simulink model "neeew"  (Simulink 8.3)
settings: Solver=ode23tb  SolverMode=SingleTasking  StartTime=0.0  StopTime=1  RelTol=1e-3
undefined symbols (not defined in the file): D1, Delta
libraries: spsThreePhaseVIMeasurementLib x15, spsPiSectionLineLib x15, spsThreePhaseBreakerLib x14, spsThreePhaseParallelRLCLoadLib x5, spsThreePhaseProgrammableVoltageSourceLib x2, spsThreePhaseTransformerTwoWindingsLib x2, spsGroundLib x2, spspowerguiLib x1
settings Model: Creator=DELL  LastModifiedBy=Ayyan LapTop  CovMetricSettings=dwe  CovHtmlReporting=off  covSaveCumulativeToWorkspaceVar=off  CovSaveSingleToWorkspaceVar=off  CovExternalEMLEnable=on  CovSFcnEnable=on
settings SolverCC: ZeroCrossAlgorithm=Adaptive
settings DataIOCC: LimitDataPoints=off  SaveFormat=StructureWithTime  SignalLoggingSaveFormat=Dataset
settings DebuggingCC: UnderspecifiedInitializationDetection=Simplified  MergeDetectMultiDrivingBlocksExec=error  MaxConsecutiveZCsMsg=none  SolverPrmCheckMsg=none  FrameProcessingCompatibilityMsg=error  StateNameClashWarn=none  SFUnexpectedBacktrackingDiag=error  SFNoUnconditionalDefaultTransitionDiag=error
settings HardwareCC: ProdBitPerPointer=64  ProdLargestAtomicFloat=Float  ProdIntDivRoundTo=Zero  ProdEndianess=LittleEndian  ProdHWDeviceType=Specified
settings ModelReferenceCC: PropagateSignalLabelsOutOfModel=on
settings GRTTargetCC: TargetLangStandard=C99 (ISO)  CombineOutputUpdateFcns=on  GRTInterface=off

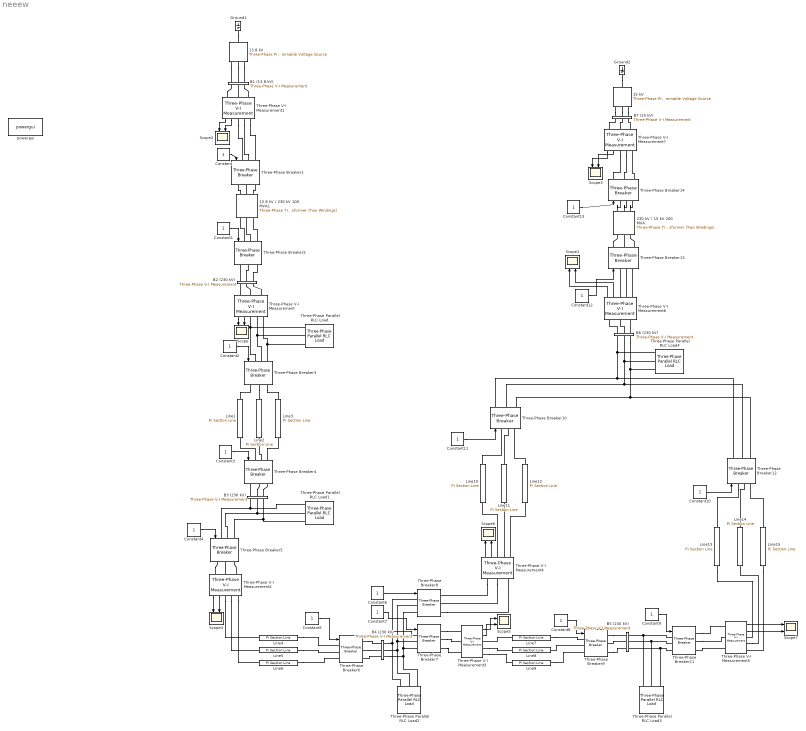
== system neeew ==
  13.8 kV : spsThreePhaseProgrammableVoltageSourceLib/Three-Phase Programmable Voltage Source  PositiveSequence=[13.8e3 0 60]  VariationEntity=Amplitude  VariationType=Table of time-amplitude pairs  VariationTypeAlt=Step  VariationStep=-0.2  VariationRate=10  VariationMagnitude=0.3  VariationFrequency=2  VariationTiming=[0.05 0.05+5/60]  VariationPhaseA=off  Amplitudes=[1 0.75 1.0]  TimeValues=[0 0.03 0.13]  HarmonicGeneration=off  HarmonicA=[1 -0.1 0 2]  HarmonicB=[2 0.15 35 2]*0  Timing="[0.1  2]"  BusType=PV  Pref=100e6  Qref=0  Qmin=-inf  Qmax=inf
  13.8 kV / 230 kV 100 MVA1 : spsThreePhaseTransformerTwoWindingsLib/Three-Phase Transformer (Two Windings)  Winding1Connection=Delta (D1)  Winding2Connection=Yg  CoreType=Three single-phase transformers  SetSaturation=off  Hysteresis=off  DataFile='basic_model'  SetInitialFlux=off  Measurements=None  UNITS=pu  NominalPower=[100e6 60 ]  Winding1="[ 13.8e3  0.1/30   0.1 ]"  Winding2="[ 230e3  0.1/30  0.1]"  Rm=500  Lm=500  L0=0.5  Saturation="[ 0,0  ;  0.005,1.2  ;  1.0,1.4 ]"  InitialFluxes=[ 0.8 , -0.8 , 0.7 ]  BreakLoop=off  DiscreteSolver=Trapezoidal iterative  DataType=off  TransfoNumber=0
  15 kV : spsThreePhaseProgrammableVoltageSourceLib/Three-Phase Programmable Voltage Source  PositiveSequence=[15e3 0 60]  VariationEntity=Amplitude  VariationType=Table of time-amplitude pairs  VariationTypeAlt=Step  VariationStep=-0.2  VariationRate=10  VariationMagnitude=0.3  VariationFrequency=2  VariationTiming=[0.05 0.05+5/60]  VariationPhaseA=off  Amplitudes=[1 0.75 1.0]  TimeValues=[0 0.03 0.13]  HarmonicGeneration=off  HarmonicA=[1 -0.1 0 2]  HarmonicB=[2 0.15 35 2]*0  Timing="[0.1  2]"  BusType=PQ  Pref=200e6  Qref=inf  Qmin=-inf  Qmax=inf
  230 kV / 15 kV 200 MVA : spsThreePhaseTransformerTwoWindingsLib/Three-Phase Transformer (Two Windings)  Winding1Connection=Delta (D1)  Winding2Connection=Yg  CoreType=Three single-phase transformers  SetSaturation=off  Hysteresis=off  DataFile='basic_model'  SetInitialFlux=off  Measurements=None  UNITS=pu  NominalPower=[200e6 60 ]  Winding1="[ 15e3  0.1/30   0.1 ]"  Winding2="[ 230e3  0.1/30  0.1]"  Rm=500  Lm=500  L0=0.5  Saturation="[ 0,0  ;  0.005,1.2  ;  1.0,1.4 ]"  InitialFluxes=[ 0.8 , -0.8 , 0.7 ]  BreakLoop=off  DiscreteSolver=Trapezoidal iterative  DataType=off  TransfoNumber=0
  B1 (13.8 kV) : spsThreePhaseVIMeasurementLib/Three-Phase V-I Measurement  VoltageMeasurement=no  SetLabelV=off  LabelV=Vabc_B120  Vpu=off  VpuLL=off  CurrentMeasurement=no  SetLabelI=on  LabelI=Iabc_B120  Ipu=off  Pbase=100e6  Vbase=120e3  OutputType=Complex  PhasorSimulation=off  PSBequivalent=0
  B2 (230 kV) : spsThreePhaseVIMeasurementLib/Three-Phase V-I Measurement  VoltageMeasurement=no  SetLabelV=off  LabelV=Vabc_B120  Vpu=off  VpuLL=off  CurrentMeasurement=no  SetLabelI=on  LabelI=Iabc_B120  Ipu=off  Pbase=100e6  Vbase=120e3  OutputType=Complex  PhasorSimulation=off  PSBequivalent=0
  B3 (230 kV) : spsThreePhaseVIMeasurementLib/Three-Phase V-I Measurement  VoltageMeasurement=no  SetLabelV=off  LabelV=Vabc_B120  Vpu=off  VpuLL=off  CurrentMeasurement=no  SetLabelI=on  LabelI=Iabc_B120  Ipu=off  Pbase=100e6  Vbase=120e3  OutputType=Complex  PhasorSimulation=off  PSBequivalent=0
  B4 (230 kV) : spsThreePhaseVIMeasurementLib/Three-Phase V-I Measurement  VoltageMeasurement=no  SetLabelV=off  LabelV=Vabc_B120  Vpu=off  VpuLL=off  CurrentMeasurement=no  SetLabelI=on  LabelI=Iabc_B120  Ipu=off  Pbase=100e6  Vbase=120e3  OutputType=Complex  PhasorSimulation=off  PSBequivalent=0
  B5 (230 kV) : spsThreePhaseVIMeasurementLib/Three-Phase V-I Measurement  VoltageMeasurement=no  SetLabelV=off  LabelV=Vabc_B120  Vpu=off  VpuLL=off  CurrentMeasurement=no  SetLabelI=on  LabelI=Iabc_B120  Ipu=off  Pbase=100e6  Vbase=120e3  OutputType=Complex  PhasorSimulation=off  PSBequivalent=0
  B6 (230 kV) : spsThreePhaseVIMeasurementLib/Three-Phase V-I Measurement  VoltageMeasurement=no  SetLabelV=off  LabelV=Vabc_B120  Vpu=off  VpuLL=off  CurrentMeasurement=no  SetLabelI=on  LabelI=Iabc_B120  Ipu=off  Pbase=100e6  Vbase=120e3  OutputType=Complex  PhasorSimulation=off  PSBequivalent=0
  B7 (15 kV) : spsThreePhaseVIMeasurementLib/Three-Phase V-I Measurement  VoltageMeasurement=no  SetLabelV=off  LabelV=Vabc_B120  Vpu=off  VpuLL=off  CurrentMeasurement=no  SetLabelI=on  LabelI=Iabc_B120  Ipu=off  Pbase=100e6  Vbase=120e3  OutputType=Complex  PhasorSimulation=off  PSBequivalent=0
  Constant{,1..13} (14 alike) : Constant
  Ground1 : spsGroundLib/Ground  LConnTagsString=a
  Ground2 : spsGroundLib/Ground  LConnTagsString=a
  Line{1..3,13..15} (6 alike) : spsPiSectionLineLib/Pi Section Line  LConnTagsString=__new0  RConnTagsString=__new0  Phases=1  PiSections=2  Length=15  Frequency=50  Resistance=.08  Inductance=.0016  Capacitance=1e-6  Measurements=None  Measurements2=None
  Line10 : spsPiSectionLineLib/Pi Section Line  LConnTagsString=__new0  RConnTagsString=__new0  Phases=1  PiSections=2  Length=50  Frequency=50  Resistance=.08  Inductance=.0016  Capacitance=1e-6  Measurements=None  Measurements2=None
  Line11 : spsPiSectionLineLib/Pi Section Line  LConnTagsString=__new0  RConnTagsString=__new0  Phases=1  PiSections=2  Length=50  Frequency=50  Resistance=.08  Inductance=.0016  Capacitance=1e-6  Measurements=None  Measurements2=None
  Line12 : spsPiSectionLineLib/Pi Section Line  LConnTagsString=__new0  RConnTagsString=__new0  Phases=1  PiSections=2  Length=50  Frequency=50  Resistance=.08  Inductance=.0016  Capacitance=1e-6  Measurements=None  Measurements2=None
  Line4 : spsPiSectionLineLib/Pi Section Line  LConnTagsString=__new0  RConnTagsString=__new0  Phases=1  PiSections=2  Length=30  Frequency=50  Resistance=.08  Inductance=.0016  Capacitance=1e-6  Measurements=None  Measurements2=None
  Line5 : spsPiSectionLineLib/Pi Section Line  LConnTagsString=__new0  RConnTagsString=__new0  Phases=1  PiSections=2  Length=30  Frequency=50  Resistance=.08  Inductance=.0016  Capacitance=1e-6  Measurements=None  Measurements2=None
  Line6 : spsPiSectionLineLib/Pi Section Line  LConnTagsString=__new0  RConnTagsString=__new0  Phases=1  PiSections=2  Length=30  Frequency=50  Resistance=.08  Inductance=.0016  Capacitance=1e-6  Measurements=None  Measurements2=None
  Line7 : spsPiSectionLineLib/Pi Section Line  LConnTagsString=__new0  RConnTagsString=__new0  Phases=1  PiSections=2  Length=40  Frequency=50  Resistance=.08  Inductance=.0016  Capacitance=1e-6  Measurements=None  Measurements2=None
  Line8 : spsPiSectionLineLib/Pi Section Line  LConnTagsString=__new0  RConnTagsString=__new0  Phases=1  PiSections=2  Length=40  Frequency=50  Resistance=.08  Inductance=.0016  Capacitance=1e-6  Measurements=None  Measurements2=None
  Line9 : spsPiSectionLineLib/Pi Section Line  LConnTagsString=__new0  RConnTagsString=__new0  Phases=1  PiSections=2  Length=40  Frequency=50  Resistance=.08  Inductance=.0016  Capacitance=1e-6  Measurements=None  Measurements2=None
  Scope{,1..7} (8 alike) : Scope  NumInputPorts=2
      Scope settings: TimeRange=auto  MaxDataPoints=5000  SaveToWorkspace=off  YMin=-5~-5  YMax=5~5  SampleTime=-1
      Scope1 settings: TimeRange=auto  MaxDataPoints=5000  SaveToWorkspace=off  SaveName=ScopeData2  YMin=-5~-5  YMax=5~5  SampleTime=-1
      Scope2 settings: TimeRange=auto  MaxDataPoints=5000  SaveToWorkspace=off  SaveName=ScopeData3  YMin=-24395.18395~-69245.32679  YMax=24395.18395~68433.69318  SampleTime=-1
      Scope3 settings: TimeRange=auto  MaxDataPoints=5000  SaveToWorkspace=off  SaveName=ScopeData4  YMin=-5~-5  YMax=5~5  SampleTime=-1
      Scope4 settings: TimeRange=auto  MaxDataPoints=5000  SaveToWorkspace=off  SaveName=ScopeData5  YMin=-5~-5  YMax=5~5  SampleTime=-1
      Scope5 settings: TimeRange=auto  MaxDataPoints=5000  SaveToWorkspace=off  SaveName=ScopeData6  YMin=-5~-5  YMax=5~5  SampleTime=-1
      Scope6 settings: TimeRange=auto  MaxDataPoints=5000  SaveToWorkspace=off  SaveName=ScopeData7  YMin=-5~-5  YMax=5~5  SampleTime=-1
      Scope7 settings: TimeRange=auto  MaxDataPoints=5000  SaveToWorkspace=off  SaveName=ScopeData  YMin=-5~-5  YMax=5~5  SampleTime=-1
  Three-Phase Breaker{1..14} (14 alike) : spsThreePhaseBreakerLib/Three-Phase Breaker  InitialState=closed  SwitchA=on  SwitchB=on  SwitchC=on  SwitchTimes="[4/60  10/60]"  External=on  BreakerResistance=0.001  SnubberResistance=1e6  SnubberCapacitance=inf  Measurements=None
  Three-Phase Parallel RLC Load{,1..4} (5 alike) : spsThreePhaseParallelRLCLoadLib/Three-Phase Parallel RLC Load  LConnTagsString=A|B|C  Configuration=Y (grounded)  NominalVoltage=230e3  Vabc=[1e3 1e3 1e3]  Vabcp=[1e3 1e3 1e3]  NominalFrequency=60  UnbalancedPower=off  ActivePower=50e3  InductivePower=30e3  CapacitivePower=0  Pabc=[10e3 9e3 11e3]  QLabc=[100 90 110]  QCabc=[100 90 110]  Pabcp=[10e3 9e3 11e3]  QLabcp=[100 90 110]  QCabcp=[100 90 110]  Measurements=None  LoadType=constant Z
  Three-Phase V-I Measurement{,1..7} (8 alike) : spsThreePhaseVIMeasurementLib/Three-Phase V-I Measurement  VoltageMeasurement=phase-to-phase  SetLabelV=off  LabelV=Vabc  Vpu=off  VpuLL=off  CurrentMeasurement=yes  SetLabelI=off  LabelI=Iabc  Ipu=off  Pbase=100e6  Vbase=500e3  OutputType=Complex  PhasorSimulation=off  PSBequivalent=0
  powergui : spspowerguiLib/powergui  Priority=1  SimulationMode=Discrete  SampleTime=50e-6  frequency=60  Iterations=50  frequencyindice=60  Pbase=100e6  ErrMax=1e-4  UnitsV=kV  UnitsW=MW  buscounter=0  FunctionMessages=off  echomessages=off  EnableUseOfTLC=off  CurrentSourceSwitches=off  DisableSnubberDevices=off  DisableRonSwitches=off  DisableVfSwitches=off  DisplayEquations=off  AutomaticDiscreteSolvers=off  SolverType=Tustin/Backward Euler (TBE)  Interpol=off  ExternalGateDelay=off  methode=off  Ts=100  x0status=blocks  SPID=on  SwTol=0  HookPort=off  NonlinearTolerance=1e-4  nMaxIteration=100  ContinueOnMaxIteration=off  RestoreLinks=warning  ResistiveCurrentMeasurement=off  Frange=[0:2:500]  Ylog=off  Xlog=on  ShowGrid=off  save=off  variable=ZData  structure=0  ZoomFFT=off  StartTime=0.0  cycles=1  DisplayStyle=1  fundamental=60  FreqAxis=off  MaxFrequency=1000  frequencyindicesteady=1  RmsSteady=1  display=off
  wires:
  Constant9/1 -> Three-Phase Breaker11/1
  Three-Phase V-I Measurement2/2 -> Scope4/2
  Constant6/1 -> Three-Phase Breaker8/1
  Constant11/1 -> Three-Phase Breaker10/1
  Constant7/1 -> Three-Phase Breaker7/1
  Constant8/1 -> Three-Phase Breaker9/1
  Constant/1 -> Three-Phase Breaker1/1
  Constant13/1 -> Three-Phase Breaker14/1
  Constant10/1 -> Three-Phase Breaker12/1
  Constant2/1 -> Three-Phase Breaker3/1
  Three-Phase V-I Measurement7/1 -> Scope3/1
  Constant4/1 -> Three-Phase Breaker5/1
  Three-Phase V-I Measurement7/2 -> Scope3/2
  Constant3/1 -> Three-Phase Breaker4/1
  Constant5/1 -> Three-Phase Breaker6/1
  Constant1/1 -> Three-Phase Breaker2/1
  Three-Phase V-I Measurement6/1 -> Scope1/1
  Three-Phase V-I Measurement5/2 -> Scope7/2
  Three-Phase V-I Measurement4/1 -> Scope6/1
  Three-Phase V-I Measurement/2 -> Scope/2
  Three-Phase V-I Measurement3/2 -> Scope5/2
  Three-Phase V-I Measurement3/1 -> Scope5/1
  Three-Phase V-I Measurement1/2 -> Scope2/2
  Three-Phase V-I Measurement2/1 -> Scope4/1
  Three-Phase V-I Measurement4/2 -> Scope6/2
  Three-Phase V-I Measurement1/1 -> Scope2/1
  Three-Phase V-I Measurement/1 -> Scope/1
  Three-Phase V-I Measurement6/2 -> Scope1/2
  Three-Phase V-I Measurement5/1 -> Scope7/1
  Constant12/1 -> Three-Phase Breaker13/1
  connections:
  B6 (230 kV)/LConn2 -- Three-Phase Parallel RLC Load4/LConn2 -- Three-Phase Breaker10/RConn2 -- Three-Phase Breaker12/RConn2
  Three-Phase Breaker8/LConn2 -- B4 (230 kV)/LConn2 -- Three-Phase Parallel RLC Load2/LConn2 -- Three-Phase Breaker7/LConn2
  B3 (230 kV)/RConn1 -- Three-Phase Breaker5/LConn1 -- Three-Phase Parallel RLC Load1/LConn1
  Three-Phase Breaker7/LConn1 -- B4 (230 kV)/LConn1 -- Three-Phase Parallel RLC Load2/LConn1 -- Three-Phase Breaker8/LConn1
  B6 (230 kV)/LConn1 -- Three-Phase Breaker10/RConn1 -- Three-Phase Breaker12/RConn1 -- Three-Phase Parallel RLC Load4/LConn1
  B5 (230 kV)/LConn3 -- Three-Phase Breaker11/LConn3 -- Three-Phase Parallel RLC Load3/LConn3
  Three-Phase Breaker12/RConn3 -- Three-Phase Breaker10/RConn3 -- B6 (230 kV)/LConn3 -- Three-Phase Parallel RLC Load4/LConn3
  B5 (230 kV)/LConn2 -- Three-Phase Breaker11/LConn2 -- Three-Phase Parallel RLC Load3/LConn2
  Three-Phase Parallel RLC Load3/LConn1 -- Three-Phase Breaker11/LConn1 -- B5 (230 kV)/LConn1
  Three-Phase V-I Measurement/RConn3 -- Three-Phase Breaker3/LConn3 -- Three-Phase Parallel RLC Load/LConn3
  Three-Phase Breaker8/LConn3 -- Three-Phase Breaker7/LConn3 -- B4 (230 kV)/LConn3 -- Three-Phase Parallel RLC Load2/LConn3
  B3 (230 kV)/RConn2 -- Three-Phase Breaker5/LConn2 -- Three-Phase Parallel RLC Load1/LConn2
  Three-Phase Breaker3/LConn1 -- Three-Phase V-I Measurement/RConn1 -- Three-Phase Parallel RLC Load/LConn1
  Three-Phase Parallel RLC Load1/LConn3 -- Three-Phase Breaker5/LConn3 -- B3 (230 kV)/RConn3
  Three-Phase Parallel RLC Load/LConn2 -- Three-Phase Breaker3/LConn2 -- Three-Phase V-I Measurement/RConn2
  Line15/LConn1 -- Three-Phase V-I Measurement5/RConn3
  Three-Phase Breaker13/RConn1 -- 230 kV / 15 kV 200 MVA/RConn1
  230 kV / 15 kV 200 MVA/LConn1 -- Three-Phase Breaker14/LConn1
  Three-Phase Breaker3/RConn2 -- Line2/LConn1
  Three-Phase V-I Measurement2/RConn2 -- Line5/LConn1
  Three-Phase Breaker10/LConn2 -- Line11/RConn1
  Three-Phase V-I Measurement1/RConn1 -- Three-Phase Breaker1/LConn1
  Three-Phase Breaker13/RConn3 -- 230 kV / 15 kV 200 MVA/RConn3
  Three-Phase Breaker3/RConn3 -- Line3/LConn1
  Three-Phase V-I Measurement2/LConn1 -- Three-Phase Breaker5/RConn1
  Three-Phase V-I Measurement4/RConn2 -- Line11/LConn1
  Three-Phase V-I Measurement2/RConn3 -- Line6/LConn1
  Three-Phase Breaker11/RConn1 -- Three-Phase V-I Measurement5/LConn1
  Three-Phase Breaker13/RConn2 -- 230 kV / 15 kV 200 MVA/RConn2
  Three-Phase Breaker9/RConn1 -- B5 (230 kV)/RConn1
  13.8 kV/RConn3 -- B1 (13.8 kV)/LConn3
  Three-Phase V-I Measurement7/LConn1 -- B7 (15 kV)/LConn1
  Three-Phase Breaker3/RConn1 -- Line1/LConn1
  Three-Phase V-I Measurement7/LConn3 -- B7 (15 kV)/LConn3
  Three-Phase Breaker4/LConn1 -- Line1/RConn1
  Three-Phase Breaker7/RConn3 -- Three-Phase V-I Measurement3/LConn3
  Three-Phase V-I Measurement4/LConn2 -- Three-Phase Breaker8/RConn2
  Line7/RConn1 -- Three-Phase Breaker9/LConn1
  Three-Phase Breaker2/LConn1 -- 13.8 kV / 230 kV 100 MVA1/RConn1
  B6 (230 kV)/RConn1 -- Three-Phase V-I Measurement6/LConn1
  Three-Phase V-I Measurement7/RConn2 -- Three-Phase Breaker14/RConn2
  Line12/RConn1 -- Three-Phase Breaker10/LConn3
  Three-Phase Breaker1/RConn1 -- 13.8 kV / 230 kV 100 MVA1/LConn1
  Three-Phase Breaker14/RConn3 -- Three-Phase V-I Measurement7/RConn3
  B3 (230 kV)/LConn3 -- Three-Phase Breaker4/RConn3
  Line4/RConn1 -- Three-Phase Breaker6/LConn1
  13.8 kV/RConn2 -- B1 (13.8 kV)/LConn2
  Three-Phase V-I Measurement1/LConn1 -- B1 (13.8 kV)/RConn1
  B2 (230 kV)/LConn1 -- Three-Phase Breaker2/RConn1
  Three-Phase V-I Measurement7/RConn1 -- Three-Phase Breaker14/RConn1
  B2 (230 kV)/LConn3 -- Three-Phase Breaker2/RConn3
  Three-Phase Breaker7/RConn1 -- Three-Phase V-I Measurement3/LConn1
  Three-Phase Breaker12/LConn1 -- Line13/RConn1
  B3 (230 kV)/LConn1 -- Three-Phase Breaker4/RConn1
  Three-Phase V-I Measurement5/RConn2 -- Line14/LConn1
  Three-Phase V-I Measurement6/RConn3 -- Three-Phase Breaker13/LConn3
  Three-Phase V-I Measurement1/LConn3 -- B1 (13.8 kV)/RConn3
  B6 (230 kV)/RConn3 -- Three-Phase V-I Measurement6/LConn3
  Three-Phase V-I Measurement4/LConn1 -- Three-Phase Breaker8/RConn1
  Three-Phase V-I Measurement4/RConn1 -- Line10/LConn1
  Three-Phase V-I Measurement/LConn1 -- B2 (230 kV)/RConn1
  Three-Phase V-I Measurement4/RConn3 -- Line12/LConn1
  Three-Phase V-I Measurement3/RConn3 -- Line9/LConn1
  Three-Phase Breaker11/RConn3 -- Three-Phase V-I Measurement5/LConn3
  Line13/LConn1 -- Three-Phase V-I Measurement5/RConn1
  Three-Phase Breaker6/RConn1 -- B4 (230 kV)/RConn1
  Three-Phase V-I Measurement3/RConn2 -- Line8/LConn1
  230 kV / 15 kV 200 MVA/LConn2 -- Three-Phase Breaker14/LConn2
  Three-Phase V-I Measurement2/LConn3 -- Three-Phase Breaker5/RConn3
  Line7/LConn1 -- Three-Phase V-I Measurement3/RConn1
  Three-Phase V-I Measurement2/LConn2 -- Three-Phase Breaker5/RConn2
  Three-Phase V-I Measurement1/RConn2 -- Three-Phase Breaker1/LConn2
  Three-Phase V-I Measurement6/RConn1 -- Three-Phase Breaker13/LConn1
  Three-Phase Breaker8/RConn3 -- Three-Phase V-I Measurement4/LConn3
  15 kV/RConn3 -- B7 (15 kV)/RConn3
  Three-Phase V-I Measurement2/RConn1 -- Line4/LConn1
  15 kV/RConn2 -- B7 (15 kV)/RConn2
  15 kV/RConn1 -- B7 (15 kV)/RConn1
  Three-Phase V-I Measurement7/LConn2 -- B7 (15 kV)/LConn2
  Ground1/LConn1 -- 13.8 kV/LConn1
  Three-Phase Breaker4/LConn3 -- Line3/RConn1
  Three-Phase Breaker2/LConn2 -- 13.8 kV / 230 kV 100 MVA1/RConn2
  Ground2/LConn1 -- 15 kV/LConn1
  Three-Phase Breaker9/RConn3 -- B5 (230 kV)/RConn3
  Line6/RConn1 -- Three-Phase Breaker6/LConn3
  Three-Phase Breaker7/RConn2 -- Three-Phase V-I Measurement3/LConn2
  Three-Phase Breaker11/RConn2 -- Three-Phase V-I Measurement5/LConn2
  Three-Phase Breaker4/LConn2 -- Line2/RConn1
  Three-Phase Breaker12/LConn2 -- Line14/RConn1
  Three-Phase V-I Measurement6/RConn2 -- Three-Phase Breaker13/LConn2
  13.8 kV/RConn1 -- B1 (13.8 kV)/LConn1
  Three-Phase V-I Measurement/LConn2 -- B2 (230 kV)/RConn2
  Line9/RConn1 -- Three-Phase Breaker9/LConn3
  Three-Phase Breaker9/RConn2 -- B5 (230 kV)/RConn2
  Line8/RConn1 -- Three-Phase Breaker9/LConn2
  Three-Phase Breaker6/RConn2 -- B4 (230 kV)/RConn2
  Three-Phase V-I Measurement1/LConn2 -- B1 (13.8 kV)/RConn2
  230 kV / 15 kV 200 MVA/LConn3 -- Three-Phase Breaker14/LConn3
  13.8 kV / 230 kV 100 MVA1/LConn2 -- Three-Phase Breaker1/RConn2
  B3 (230 kV)/LConn2 -- Three-Phase Breaker4/RConn2
  Line5/RConn1 -- Three-Phase Breaker6/LConn2
  Three-Phase Breaker1/RConn3 -- 13.8 kV / 230 kV 100 MVA1/LConn3
  Line10/RConn1 -- Three-Phase Breaker10/LConn1
  Three-Phase V-I Measurement1/RConn3 -- Three-Phase Breaker1/LConn3
  B6 (230 kV)/RConn2 -- Three-Phase V-I Measurement6/LConn2
  B2 (230 kV)/LConn2 -- Three-Phase Breaker2/RConn2
  Three-Phase Breaker2/LConn3 -- 13.8 kV / 230 kV 100 MVA1/RConn3
  Three-Phase Breaker6/RConn3 -- B4 (230 kV)/RConn3
  Line15/RConn1 -- Three-Phase Breaker12/LConn3
  Three-Phase V-I Measurement/LConn3 -- B2 (230 kV)/RConn3
